simulink model "simu"  (R2016a)
settings: Solver=VariableStepAuto  StartTime=0.0  StopTime=10.0  RelTol=1e-3
settings Model: Creator=Eunice  LastModifiedBy=Eunice

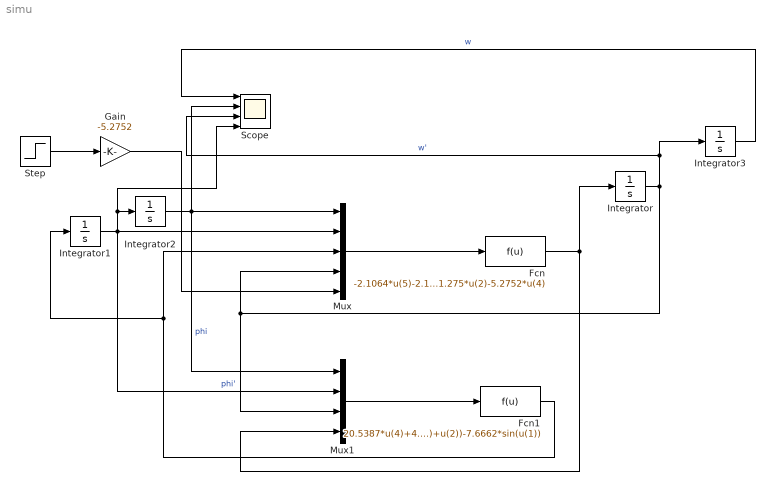
== system simu ==
  Fcn : Fcn  Expr=-2.1064*u(5)-2.1831*u(3)+5.2418*2*cos(u(1))*u(3)-5.2418*sin(2*u(1))*(1/cos(u(1)))*u(2)-151.275*u(2)-5.2752*u(4)
  Fcn1 : Fcn  Expr=20.5387*u(4)+4.6832*cos(u(1))*u(4)+3.0437*(u(3)+u(2))-7.6662*sin(u(1))
  Gain : Gain  Gain=-5.2752
  Integrator{,1..3} (4 alike) : Integrator
  Mux : Mux  Inputs=5
  Mux1 : Mux
  Scope : Scope  NumInputPorts=4
  Step : Step  After=87  SampleTime=0
  wires:
  Mux/1 -> Fcn/1
  Mux1/1 -> Fcn1/1
  Fcn/1 -> Integrator/1, Mux1/4
  Integrator/1 -> Integrator3/1, Scope/3, Mux/4, Mux1/3  "w'"
  Fcn1/1 -> Integrator1/1, Mux/3
  Integrator1/1 -> Mux1/2, Scope/4, Integrator2/1, Mux/2  "phi'"
  Integrator2/1 -> Scope/2, Mux1/1, Mux/1  "phi"
  Integrator3/1 -> Scope/1  "w"
  Gain/1 -> Mux/5
  Step/1 -> Gain/1
